simulink model "failureInputReadVtolTailsitter"  (R2026a)
settings: configuration reference "standardSILConfiguraitonParams" (kept outside this file)
undefined symbols (not defined in the file or in its folder): EnumHexFailureType, opts
libraries: simulink x3
settings Model: Creator=Edison Altamirano  LastModifiedBy=Edison Altamirano
settings ConfigSetRef: SourceName=standardSILConfiguraitonParams  SourceLocation=Base Workspace

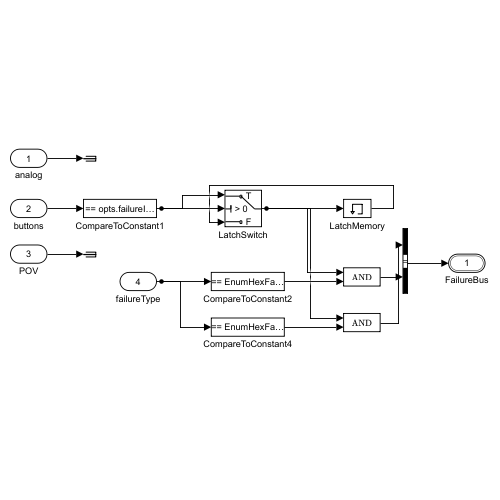
[thumbnail: Simulink's stored preview of the top-level diagram]
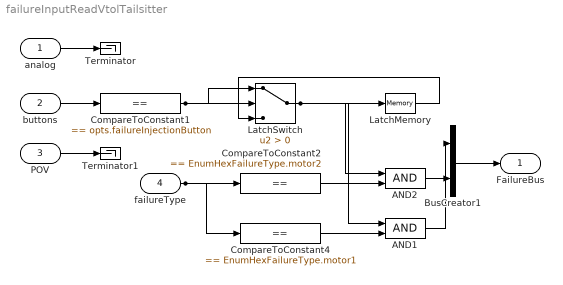
== system failureInputReadVtolTailsitter ==
  analog : Inport  PortDimensions=6
  buttons : Inport  Port=2  OutDataTypeStr=uint32
  POV : Inport  Port=3
  failureType : Inport  Port=4  OutDataTypeStr=Enum: EnumHexFailureType
  AND1 : Logic  AllPortsSameDT=off  OutDataTypeStr=boolean
  AND2 : Logic  AllPortsSameDT=off  OutDataTypeStr=boolean
  BusCreator1 : BusCreator  Inputs=2  OutDataTypeStr=Bus: FailureBus
  CompareToConstant1 : simulink/Logic and Bit Operations/Compare To Constant  relop===  const=opts.failureInjectionButton  OutDataTypeStr=boolean
  CompareToConstant2 : simulink/Logic and Bit Operations/Compare To Constant  relop===  const=EnumHexFailureType.motor2  OutDataTypeStr=boolean
  CompareToConstant4 : simulink/Logic and Bit Operations/Compare To Constant  relop===  const=EnumHexFailureType.motor1  OutDataTypeStr=boolean
  LatchMemory : Memory
  LatchSwitch : Switch  Criteria=u2 > Threshold  SaturateOnIntegerOverflow=off  InputSameDT=off
  Terminator : Terminator
  Terminator1 : Terminator
  FailureBus : Outport  OutDataTypeStr=Bus: FailureBus
  wires:
  analog/1 -> Terminator/1
  failureType/1 -> CompareToConstant4/1, CompareToConstant2/1
  buttons/1 -> CompareToConstant1/1
  CompareToConstant1/1 -> LatchSwitch/1, LatchSwitch/2
  POV/1 -> Terminator1/1
  LatchSwitch/1 -> LatchMemory/1, AND2/1, AND1/1
  CompareToConstant2/1 -> AND2/2
  CompareToConstant4/1 -> AND1/2
  LatchMemory/1 -> LatchSwitch/3
  AND2/1 -> BusCreator1/2
  AND1/1 -> BusCreator1/1
  BusCreator1/1 -> FailureBus/1
